simulink model "ControlledResistor_mod_7b"  (Simulink 7.0)
settings: Solver=ode3  StartTime=0.0  StopTime=10.0  FixedStep=Ts  RelTol=1e-3
InitFcn:
  | Ts=0.01;
libraries: powerlib x6
settings Model: Creator=ihalatci  LastModifiedBy=ihalatci
settings DebuggingCC: SaveWithParameterizedLinksMsg=none  SignalResolutionControl=TryResolveAllWithWarning  MultiTaskDSMMsg=warning  MultiTaskCondExecSysMsg=none  StrictBusMsg=None
settings RTWCC: IncludeERTFirstTime=on
settings GRTTargetCC: TargetFcnLib=ansi_tfl_tmw.mat

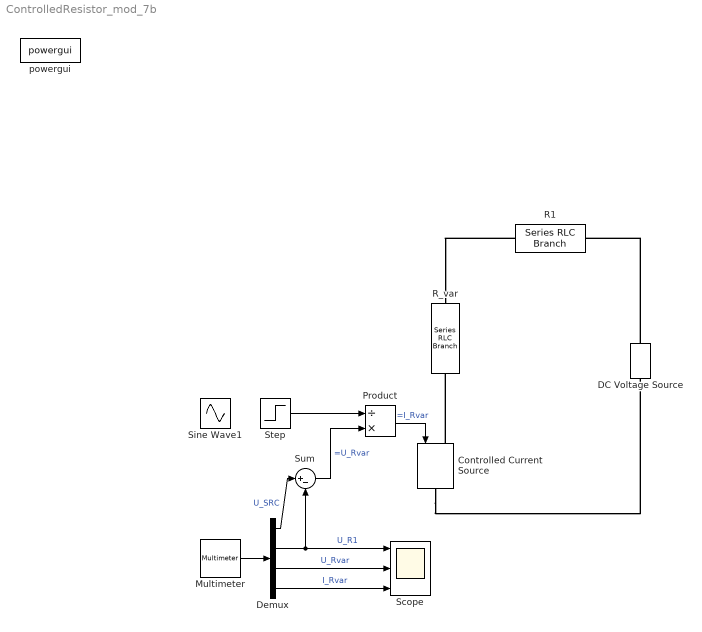
== system ControlledResistor_mod_7b ==
  Controlled Current Source : powerlib/Electrical Sources/Controlled Current Source  Orientation=down  DialogController=POWERSYS.PowerSysDialog  SystemSampleTime=-1  Initialize=on  Source_Type=DC  Amplitude=1  Phase=0  Frequency=0  Measurements=Current
  DC Voltage Source : powerlib/Electrical Sources/DC Voltage Source  Orientation=up  DialogController=POWERSYS.PowerSysDialog  SystemSampleTime=-1  Amplitude=100  Measurements=Voltage
  Demux : Demux
  Multimeter : powerlib/Measurements/Multimeter  SystemSampleTime=-1  PhasorSimulation=off  OutputType=Complex  sel=[3 2 1 4]  L=5  Gain=[1 1 1 1]  yselected={'Usrc: DC Voltage Source','Ub: R1','Ub: R_var','Ib: R_var'};  PSBOutputType=1  PSBequivalent=0  AxesSetting=[0,0.1,-100,100]  Display=0  SavedBlockNames=-11
  Product : Product  Inputs=/*  OutDataType=sfix(16)  OutScaling=2^0  RndMeth=Zero
  R1 : powerlib/Elements/Series RLC Branch  Orientation=left  DialogController=POWERSYS.PowerSysDialog  PhysicalDomain=powersysdomain  SubClassName=unknown  LeftPortType=p1  RightPortType=p1  LConnTagsString=__new0  RConnTagsString=__new0  BranchType=R  Resistance=100  Inductance=1.0  SetiL0=off  InitialCurrent=0  Capacitance=1.0  Setx0=off  InitialVoltage=0  Measurements=Branch voltage
  R_var : powerlib/Elements/Series RLC Branch  Orientation=down  DialogController=POWERSYS.PowerSysDialog  PhysicalDomain=powersysdomain  SubClassName=unknown  LeftPortType=p1  RightPortType=p1  LConnTagsString=__new0  RConnTagsString=__new0  BranchType=R  Resistance=100  Inductance=1.0  SetiL0=off  InitialCurrent=0  Capacitance=1.0  Setx0=off  InitialVoltage=0  Measurements=Branch voltage and current
  Scope : Scope  NumInputPorts=3
      settings: YMin=-5~-5~-5  YMax=5~5~5
  Sine Wave1 : Sin  Amplitude=10  Bias=11  Phase=-pi/2  SampleTime=0
  Step : Step  Time=5  Before=100  After=900  SampleTime=0
  Sum : Sum  Inputs=|+-  OutDataType=sfix(16)  OutScaling=2^0
  powergui : powerlib/powergui  SystemSampleTime=-1  SimulationMode=Discrete  SampleTime=Ts  echomessages=off  RestoreLinks=warning  x0status=blocks  Frange=[0:2:500]  Ylog=off  Xlog=on  ShowGrid=off  save=off  variable=ZData  ZoomFFT=on  StartTime=0.0  cycles=1  DisplayStyle=1  fundamental=60  FreqAxis=off  MaxFrequency=1000  frequencyindice=0  frequencyindicesteady=1  RmsSteady=1  display=off  Ts=0  frequency=60  methode=off  HookPort=off  Interpol=off  SPID=off  FunctionMessages=off
  wires:
  Product/1 -> Controlled Current Source/1  "=I_Rvar"
  Step/1 -> Product/1
  Multimeter/1 -> Demux/1
  Sum/1 -> Product/2  "=U_Rvar"
  Demux/1 -> Sum/1  "U_SRC"
  Demux/2 -> Sum/2, Scope/1  "U_R1"
  Demux/3 -> Scope/2  "U_Rvar"
  Demux/4 -> Scope/3  "I_Rvar"
  connections:
  Controlled Current Source/RConn1 -- DC Voltage Source/LConn1
  DC Voltage Source/RConn1 -- R1/LConn1
  Controlled Current Source/LConn1 -- R_var/RConn1
  R1/RConn1 -- R_var/LConn1
